simulink model "ROSCO"  (R2022b)
settings: Solver=ode4  StartTime=0.0  StopTime=TMax  FixedStep=simu.dt  RelTol=1e-3  EnableMultiTasking=on
undefined symbols (not defined in the file): DiscIntNeverNeededParam, F, OutList, Parameter, R, rpm2radps, simu, strmatch
libraries: simulink x10
(part 3 of 3)

== matlab function ROSCO/Cyclic Pitch controller/1P Cyclic Pitch Controller1/saturation (limit schedule)1 ==
  data: bdq_unsat input size=[2 1]; bdq output; b_avg input; M0 input; minPitch input; k output; Params input
%limit b_d and b_q so b_1,2,or3 does not get bigger than b_avg (the sinusoids don't get cut off at zero)
%unless b_avg is <0, then limit to 0
%at_limit is 1 if limited, 0 otherwise

function [bdq,k]  = fcn(bdq_unsat, b_avg, M0,minPitch,Params)

MODE    = Params(1);  % 1 no IPC below rated (no power loss), 2 IPC always on, 3 depends on mean load
M0_set  = Params(2);
k_sat   = Params(3);

if MODE == 1
    
    if (b_avg <= minPitch)
        bdq=[0;0];
        k = 0;
    else
        if (norm(bdq_unsat,2) <= b_avg - minPitch)
            bdq = bdq_unsat;
            k = 1;
        else
            bdq=bdq_unsat*((b_avg-minPitch)/norm(bdq_unsat,2));
            k = (b_avg/norm(bdq_unsat,2));
        end
    end
elseif MODE == 2
    if (norm(bdq_unsat,2) > deg2rad(15))
        bdq = bdq_unsat*(deg2rad(15)/norm(bdq_unsat,2));
        k = (deg2rad(15)/norm(bdq_unsat,2));
    else
        bdq = bdq_unsat;
        k = 1;
    end
else  % MODE 3
    if (M0 > M0_set - 1/(2*k_sat))
        if (M0 > M0_set + 1/(2*k_sat))
            bdq = bdq_unsat;
            k = 1;
        else
            k = k_sat*(M0-M0_set)+1/2;
            bdq = k*bdq_unsat;
        end
    else
        bdq = [0;0];
        k = 0;
    end
end
%
% if (b_avg <=0)
%         bdq = bdq_unsat;
% else
%     if (norm(bdq_unsat,2) <= b_avg)
%         bdq = bdq_unsat;
%     else
%         bdq = bdq_unsat;
%     end
% end

== matlab function ROSCO/Cyclic Pitch controller/2P Cyclic Pitch Controller2/Lead Correction ==
  data: bdq input; b_cos output size=1; psi_o input; b_sin output size=1
function [b_cos,b_sin] = fcn(bdq, psi_o)
% This block supports the Embedded MATLAB subset.
% See the help menu for details. 

b_cos=[cosd(psi_o) sind(psi_o)]*bdq;
b_sin=[-sind(psi_o) cosd(psi_o)]*bdq;

== matlab function ROSCO/Cyclic Pitch controller/2P Cyclic Pitch Controller2/d-q transformation ==
  data: RootMyb input; M_tilt output; Az input; M_yaw output; NumBl input
function [M_tilt,M_yaw] = fwdMBC2(RootMyb, Az, NumBl)
% This block supports the Embedded MATLAB subset.
% See the help menu for details.

if NumBl == 2
    
    My=RootMyb-mean(RootMyb(1:2)); %remove mean
    
    M_tilt = [cosd(2*Az) cosd(2*(Az+180)) 0]*My;
    M_yaw =  [sind(2*Az) sind(2*(Az+180)) 0]*My;
else
    My=RootMyb-mean(RootMyb); %remove mean
    
    M_tilt = [cosd(2*Az) cosd(2*(Az+120)) cosd(2*(Az+240))]*My;
    M_yaw =  [sind(2*Az) sind(2*(Az+120)) sind(2*(Az+240))]*My;
end

== matlab function ROSCO/Cyclic Pitch controller/2P Cyclic Pitch Controller2/inverse d-q transformation ==
  data: bdq input; b1 output size=1; Az input; b2 output size=1; NumBl input; b3 output size=1
function [b1,b2,b3] = bckMBC2(bdq, Az, NumBl)
% This block supports the Embedded MATLAB subset.
% See the help menu for details.


if NumBl == 2
    
    b1=[cosd(2*Az) sind(2*Az)]*bdq;
    b2=[cosd(2*(Az - 180)) sind(2*(Az - 180))]*bdq;
    b3=0;
    
else
    b1=[cosd(2*Az) sind(2*Az)]*bdq;
    b2=[cosd(2*(Az + 120)) sind(2*(Az + 120))]*bdq;
    b3=[cosd(2*(Az + 240)) sind(2*(Az + 240))]*bdq;
    
end

== matlab function ROSCO/Cyclic Pitch controller/2P Cyclic Pitch Controller2/saturation (limit schedule)1 ==
  data: bdq_unsat input size=[2 1]; bdq output; b_avg input; M0 input; minPitch input; k output; Params input
%limit b_d and b_q so b_1,2,or3 does not get bigger than b_avg (the sinusoids don't get cut off at zero)
%unless b_avg is <0, then limit to 0
%at_limit is 1 if limited, 0 otherwise

function [bdq,k]  = fcn(bdq_unsat, b_avg, M0,minPitch,Params)

MODE    = Params(1);  % 1 no IPC below rated (no power loss), 2 IPC always on, 3
M0_set  = Params(2);
k_sat   = Params(3);

if MODE == 1
    
    if (b_avg <= minPitch)
        bdq=[0;0];
        k = 0;
    else
        if (norm(bdq_unsat,2) <= b_avg - minPitch)
            bdq = bdq_unsat;
            k = 1;
        else
            bdq=bdq_unsat*((b_avg-minPitch)/norm(bdq_unsat,2));
            k = (b_avg/norm(bdq_unsat,2));
        end
    end
elseif MODE == 2
    if (norm(bdq_unsat,2) > deg2rad(15))
        bdq = bdq_unsat*(deg2rad(15)/norm(bdq_unsat,2));
        k = (deg2rad(15)/norm(bdq_unsat,2));
    else
        bdq = bdq_unsat;
        k = 1;
    end
else  % MODE 3
    if (M0 > M0_set - 1/(2*k_sat))
        if (M0 > M0_set + 1/(2*k_sat))
            bdq = bdq_unsat;
            k = 1;
        else
            k = k_sat*(M0-M0_set)+1/2;
            bdq = k*bdq_unsat;
        end
    else
        bdq = [0;0];
        k = 0;
    end
end
%
% if (b_avg <=0)
%         bdq = bdq_unsat;
% else
%     if (norm(bdq_unsat,2) <= b_avg)
%         bdq = bdq_unsat;
%     else
%         bdq = bdq_unsat;
%     end
% end

== matlab function ROSCO/Wind Speed Estimator/NaN break ==
  data: u input; y output
function y = fcn(u)

if isnan(u)
    a = 1;
end

y = u;

== matlab function ROSCO/Wind Speed Estimator/MATLAB Function ==
  settings: updateMethod=DISCRETE  sampleTime=simu.dt
  data: omega_r input; tau_g input; beta input; WE_params input; A_op input; vh output; xh input; P input; K input; xh output; P output; K output; dt input; t input; HorWind input; Cx parameter; Debug output
function [vh,xh,P,K,Debug] = WSE_EKF(omega_r, tau_g, beta, WE_params, A_op, xh,P,K,dt,t,HorWind, Cx)
% This function defines a WSE based off of an Extended Kalman Filter
% Inputs:
% Outputs:
% Nikhar Abbas

% Load R variables
J       = WE_params(1);                    % Rotor Inertia
rho     = WE_params(2);                % Air density
Rr      = WE_params(3);             % Rotor Radius, R
Ng      = WE_params(4);             % Gearbox Ratio

% Simulink Offset, between mean wind speeds due to poor startup transients
sOff    = 0.8;

% Constants
H       = [1 0 0];
R       = 0.02;
L       = 6 * Rr;
Ti      = 0.2;
A       = pi*Rr^2;                         % Rotor Swept Area, m^2


% organize Inputs
if t < dt
    om_r    = omega_r;
    v_t     = 0;
    v_m     = HorWind + sOff;
else
    om_r    = xh(1);
    v_t     = xh(2);
    v_m     = xh(3) + sOff;
end

om_m    = omega_r;

% Debug Outs
Debug   = zeros(2,1);

% Find current estimated operating conditions, and saturate
v_r     = v_t + v_m;
lambda  = om_m * Rr / v_r;
lambda  = max( min(lambda, Cx.TSR(end)), Cx.TSR(1));


% A_op (system pole) interpolation
% A_op    = interp1(R.WE_FOPoles_v,R.WE_FOPoles,xh(1) + xh(2));


% Cp interpolation
Cp      = interp2(Cx.BlPitch,Cx.TSR,Cx.Cpmat,beta * rad2deg(1),lambda);
Cp      = max(0,Cp);


% Calculate Jacobians
F       = zeros(3,3);

F(1,1)      = A_op;
F(1,2)      = 1/(2*J)*rho*A*Cp*3*(v_m+v_t)^2*1/om_r;
F(1,3)      = 1/(2*J)*rho*A*Cp*3*(v_m+v_t)^2*1/om_r;

F(2,2)      = pi * v_m / (2*L);
F(2,3)      = pi * v_t / (2*L);  % this was 0


% Calculate Covariance
Q           = zeros(3,3);
Q(1,1)      = 1e-5;                     %in DZ WSE, 1e-6
Q(2,2)      = pi * v_m^3 * Ti^2 / L;
Q(3,3)      = 2^2/600;


%% Prediction Update

% states
tau_r       = 1/2 * rho * A * Cp * v_r^3 / om_m;       % Torque calculation
tau_r       = max(tau_r,0);
a           = pi * v_m / (2 * L);                           % Wind variance
dom_r       = 1/J * (tau_r - Ng * tau_g);
dv_t        = -a*v_t;
dv_m        = 0;
dxh         = [dom_r; dv_t; dv_m];

% forward euler
xh          = xh + dt*dxh;

% covariance
dP          = F*P + P*F' + Q - K*R*K';
P           = P + dt*dP;

% kalman gain
S           = H*P*H' + R;
K           = P * H' / S(1,1);   %DZ: this is odd, keep an eye on
% K           = P * H' * inv(S);   %DZ: this is odd, keep an eye on...was probably giving NJA stability issues

% output residual & update
y_til       = om_m - om_r;
xh          = xh + K*y_til;
P           = (eye(3) - K * H) * P;         % DZ: this is also different, but I think I've seen this form before


% Output Wind Speed Estimate
vh = v_m + v_t;

% Set Debug Outputs
Debug(1) = Cp;
Debug(2) = v_m;
end

== matlab function ROSCO/Wind Speed Estimator/Soft Start ==
  settings: updateMethod=DISCRETE  sampleTime=simu.dt
  data: startTime input; out output; endTime input; time input; generic input; actual input
function out = softStart(startTime,endTime,time,generic,actual)

as  = Af_sigma(startTime,endTime);
T   = [time^3,time^2,time,1]';

if time < startTime
    act = 0;
    gen = 1;
elseif time >= startTime && time < endTime
    act = as * T; 
    gen = 1 - as * T;
else
    act = 1;
    gen = 0;
end

out = act*actual + gen*generic;

== matlab function ROSCO/PitchSaturation/Variable Saturator1 ==
  data: pitchCommand input; lowerLimit input; pitchCommandOut output; upperLimit input; atLimit output
function [pitchCommandOut,atLimit] = variableSat(pitchCommand,lowerLimit,upperLimit)
%#codegen

if pitchCommand < lowerLimit
    pitchCommandOut = lowerLimit;
    atLimit          = 1;
    
elseif pitchCommand > upperLimit
    pitchCommandOut = upperLimit;
    atLimit         = 1;
    
else
    pitchCommandOut = pitchCommand;
    atLimit         = 0;
end

== matlab function ROSCO/BldPitch Controller/Pitch GS ==
  data: Ki output size=1; Beta input; Kp_pc input; Kp output size=1; Ki_pc input; PC_beta input
function [Ki, Kp] = GainSchedule(Beta, Kp_pc, Ki_pc,  PC_beta)

% This function calculates the current gains for a Collective Blade Pitch 
% controller
%
% Inputs: v - Current wind speed estimate, m/s.
%         ContParam - Structure of control parameters, output from
%                     ControlParameters.m
%
% Outputs: Kp - Proportional Gain
%          Ki - Integral Gain
%
% Nikhar Abbas - May 2019


%% Linear Gain Schedule
% pKp_pc = ContParam.GS.pKp_pc;
% pKi_pc = ContParam.GS.pKi_pc;
% 
% %%
% Kp = pKp_pc(1)*Beta + pKp_pc(2);
% Ki = pKi_pc(1)*Beta + pKi_pc(2);
% % Kp = pKp_pc(1)*v + pKp_pc(2)
% % Ki = pKi_pc(1)*v + pKi_pc(2);
% 
% Kpmax = pKp_pc(1)*15*pi/180 + pKp_pc(2);
% Kimax = pKi_pc(1)*15*pi/180 + pKi_pc(2);
% 
% Kp = min(Kp, Kpmax);
% Ki = min(Ki,Kimax);

%% nonlinear Gain Schedule
% Kp_pc   = R.PC_GS_KP;
% Ki_pc   = R.PC_GS_KI;
% PC_beta = R.PC_GS_angles;

beta    = max(min(Beta,PC_beta(end)), PC_beta(1));

% gains
Kp      = interp1(PC_beta,Kp_pc, beta);
Ki      = interp1(PC_beta,Ki_pc, beta);



end

== matlab function ROSCO/Cyclic Pitch controller/1P Cyclic Pitch Controller1/Lead Correction ==
  data: bdq input; b_cos output size=1; psi_o input; b_sin output size=1
function [b_cos,b_sin] = fcn(bdq, psi_o)
% This block supports the Embedded MATLAB subset.
% See the help menu for details. 

b_cos=[cosd(psi_o) sind(psi_o)]*bdq;
b_sin=[-sind(psi_o) cosd(psi_o)]*bdq;
